simulink model "leftshift"  (R2024a)
settings: Solver=VariableStepAuto  StartTime=0.0  StopTime=10.0  RelTol=1e-3
libraries: simulink_extras x5
settings Model: Creator=prath  LastModifiedBy=prath

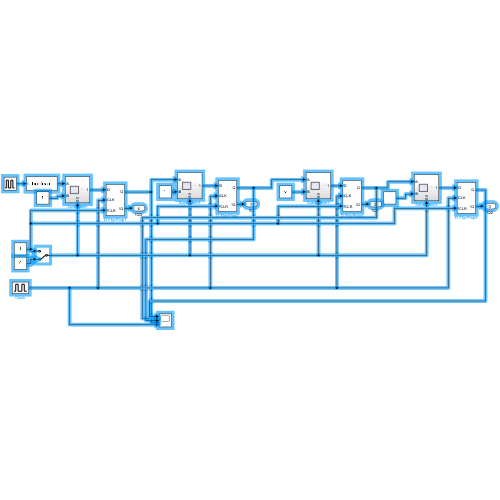
[thumbnail: Simulink's stored preview of the top-level diagram]
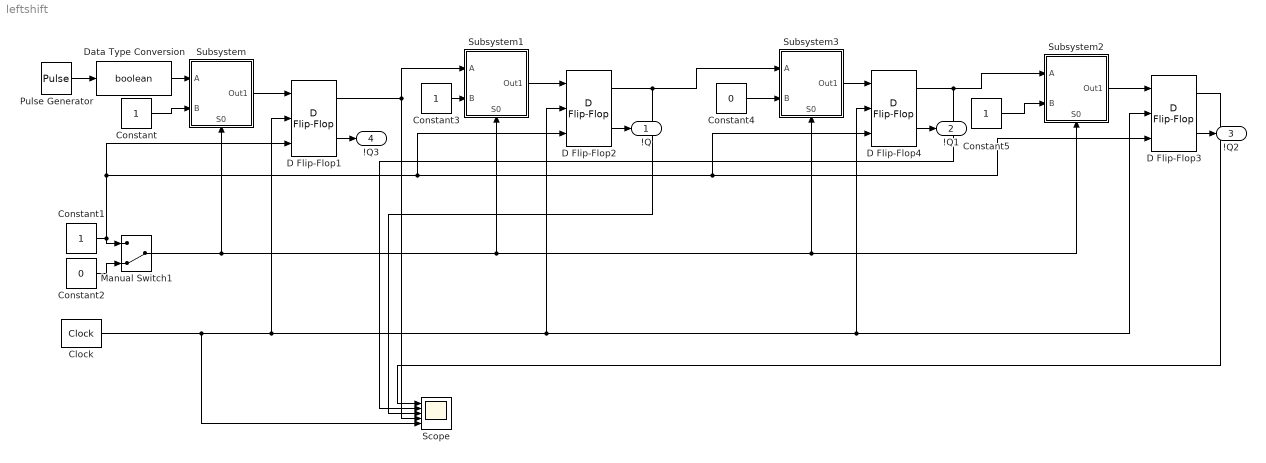
== system leftshift ==
  Clock : simulink_extras/Flip Flops/Clock  period=1
  Constant : Constant
  Constant1 : Constant  OutDataTypeStr=boolean
  Constant2 : Constant  Value=0  OutDataTypeStr=boolean
  Constant3 : Constant  OutDataTypeStr=boolean
  Constant4 : Constant  Value=0  OutDataTypeStr=boolean
  Constant5 : Constant  OutDataTypeStr=boolean
  D Flip-Flop{1..4} (4 alike) : simulink_extras/Flip Flops/D Flip-Flop
  Data Type Conversion : DataTypeConversion  OutDataTypeStr=boolean  SaturateOnIntegerOverflow=off  RndMeth=Floor
  Manual Switch1 : ManualSwitch  CurrentSetting=0
  Pulse Generator : DiscretePulseGenerator  PulseType=Time based  PulseWidth=50
  Scope : Scope  NumInputPorts=5
  Subsystem : Subsystem
      settings: PortSchema="{\"entries\":[{\"content\":{\"sides\":[{\"content\":{\"connectorIds\":[\"In1\",\"In2\"]},\"type\":\"ConnectorPlacement.EquallySpacedRectSide\",\"uuid\":\"2b5babe2-2f8b-4255-a93c-442313dac02f\"},{\"content\":{\"connectorIds\":[\"Out1\"],\"side\":\"RIGHT\"},\"type\":\"ConnectorPlacement.EquallySpacedRectSide\",\"uuid\":\"d00cf0b8-9821-435f-8e0a-21d3f86eeeec\"},{\"content\":{\"side\":\"TOP\"},\"type\":\"ConnectorPlacement.EquallySpacedRectSide\",\"uuid\":\"aded218e-ad72-4b70-8373-6f3260b36647\"},{\"content\":{\"connectorIds\":[\"In3\"],\"side\":\"BOTTOM\"},\"type\":\"ConnectorPlacement.EquallySpacedRectSide\",\"uuid\":\"ccb2f48e-c23e-4309-aab1-41b35e60905c\"}]},\"type\":\"ConnectorPlacement.EquallySpacedConnector\",\"uuid\":\"f3540823-2819-4903-8dd7-ac751c0ceac7\"}],\"packageUris\":[\"http://schema.mathworks.com/mf0/Connector/R2020b\"],\"version\":\"1.0\"}"
  Subsystem1 : Subsystem
      settings: PortSchema="{\"entries\":[{\"content\":{\"sides\":[{\"content\":{\"connectorIds\":[\"In1\",\"In2\"]},\"type\":\"ConnectorPlacement.EquallySpacedRectSide\",\"uuid\":\"2b5babe2-2f8b-4255-a93c-442313dac02f\"},{\"content\":{\"connectorIds\":[\"Out1\"],\"side\":\"RIGHT\"},\"type\":\"ConnectorPlacement.EquallySpacedRectSide\",\"uuid\":\"d00cf0b8-9821-435f-8e0a-21d3f86eeeec\"},{\"content\":{\"side\":\"TOP\"},\"type\":\"ConnectorPlacement.EquallySpacedRectSide\",\"uuid\":\"aded218e-ad72-4b70-8373-6f3260b36647\"},{\"content\":{\"connectorIds\":[\"In3\"],\"side\":\"BOTTOM\"},\"type\":\"ConnectorPlacement.EquallySpacedRectSide\",\"uuid\":\"ccb2f48e-c23e-4309-aab1-41b35e60905c\"}]},\"type\":\"ConnectorPlacement.EquallySpacedConnector\",\"uuid\":\"f3540823-2819-4903-8dd7-ac751c0ceac7\"}],\"packageUris\":[\"http://schema.mathworks.com/mf0/Connector/R2020b\"],\"version\":\"1.0\"}"
  Subsystem2 : Subsystem
      settings: PortSchema="{\"entries\":[{\"content\":{\"sides\":[{\"content\":{\"connectorIds\":[\"In1\",\"In2\"]},\"type\":\"ConnectorPlacement.EquallySpacedRectSide\",\"uuid\":\"2b5babe2-2f8b-4255-a93c-442313dac02f\"},{\"content\":{\"connectorIds\":[\"Out1\"],\"side\":\"RIGHT\"},\"type\":\"ConnectorPlacement.EquallySpacedRectSide\",\"uuid\":\"d00cf0b8-9821-435f-8e0a-21d3f86eeeec\"},{\"content\":{\"side\":\"TOP\"},\"type\":\"ConnectorPlacement.EquallySpacedRectSide\",\"uuid\":\"aded218e-ad72-4b70-8373-6f3260b36647\"},{\"content\":{\"connectorIds\":[\"In3\"],\"side\":\"BOTTOM\"},\"type\":\"ConnectorPlacement.EquallySpacedRectSide\",\"uuid\":\"ccb2f48e-c23e-4309-aab1-41b35e60905c\"}]},\"type\":\"ConnectorPlacement.EquallySpacedConnector\",\"uuid\":\"f3540823-2819-4903-8dd7-ac751c0ceac7\"}],\"packageUris\":[\"http://schema.mathworks.com/mf0/Connector/R2020b\"],\"version\":\"1.0\"}"
  Subsystem3 : Subsystem
      settings: PortSchema="{\"entries\":[{\"content\":{\"sides\":[{\"content\":{\"connectorIds\":[\"In1\",\"In2\"]},\"type\":\"ConnectorPlacement.EquallySpacedRectSide\",\"uuid\":\"2b5babe2-2f8b-4255-a93c-442313dac02f\"},{\"content\":{\"connectorIds\":[\"Out1\"],\"side\":\"RIGHT\"},\"type\":\"ConnectorPlacement.EquallySpacedRectSide\",\"uuid\":\"d00cf0b8-9821-435f-8e0a-21d3f86eeeec\"},{\"content\":{\"side\":\"TOP\"},\"type\":\"ConnectorPlacement.EquallySpacedRectSide\",\"uuid\":\"aded218e-ad72-4b70-8373-6f3260b36647\"},{\"content\":{\"connectorIds\":[\"In3\"],\"side\":\"BOTTOM\"},\"type\":\"ConnectorPlacement.EquallySpacedRectSide\",\"uuid\":\"ccb2f48e-c23e-4309-aab1-41b35e60905c\"}]},\"type\":\"ConnectorPlacement.EquallySpacedConnector\",\"uuid\":\"f3540823-2819-4903-8dd7-ac751c0ceac7\"}],\"packageUris\":[\"http://schema.mathworks.com/mf0/Connector/R2020b\"],\"version\":\"1.0\"}"
  !Q : Outport
  !Q1 : Outport  Port=2
  !Q2 : Outport  Port=3
  !Q3 : Outport  Port=4
  wires:
  D Flip-Flop1/2 -> !Q3/1
  D Flip-Flop3/2 -> !Q2/1
  D Flip-Flop4/1 -> Scope/2, Subsystem2/1(A)
  Constant4/1 -> Subsystem3/2(B)
  Clock/1 -> Scope/5, D Flip-Flop3/2, D Flip-Flop4/2, D Flip-Flop2/2, D Flip-Flop1/2
  D Flip-Flop4/2 -> !Q1/1
  Data Type Conversion/1 -> Subsystem/1(A)
  Subsystem1/1(Out1) -> D Flip-Flop2/1
  D Flip-Flop2/2 -> !Q/1
  D Flip-Flop1/1 -> Scope/4, Subsystem1/1(A)
  Subsystem2/1(Out1) -> D Flip-Flop3/1
  Constant3/1 -> Subsystem1/2(B)
  Subsystem3/1(Out1) -> D Flip-Flop4/1
  Pulse Generator/1 -> Data Type Conversion/1
  Constant/1 -> Subsystem/2(B)
  Manual Switch1/1 -> Subsystem2/3(S0), Subsystem3/3(S0), Subsystem1/3(S0), Subsystem/3(S0)
  Constant5/1 -> Subsystem2/2(B)
  D Flip-Flop2/1 -> Scope/3, Subsystem3/1(A)
  D Flip-Flop3/1 -> Scope/1
  Subsystem/1(Out1) -> D Flip-Flop1/1
  Constant1/1 -> D Flip-Flop3/3, D Flip-Flop4/3, D Flip-Flop2/3, D Flip-Flop1/3, Manual Switch1/1
  Constant2/1 -> Manual Switch1/2

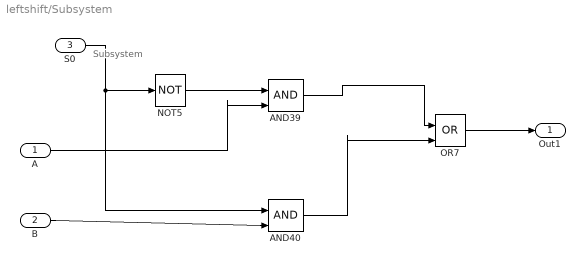
== system leftshift/Subsystem ==
  note: Subsystem
  A : Inport
  B : Inport  Port=2
  S0 : Inport  Port=3
  AND39 : Logic  IconShape=distinctive  AllPortsSameDT=off  OutDataTypeStr=boolean
  AND40 : Logic  IconShape=distinctive  AllPortsSameDT=off  OutDataTypeStr=boolean
  NOT5 : Logic  Operator=NOT  IconShape=distinctive  AllPortsSameDT=off  OutDataTypeStr=boolean
  OR7 : Logic  Operator=OR  IconShape=distinctive  AllPortsSameDT=off  OutDataTypeStr=boolean
  Out1 : Outport
  wires:
  A/1 -> AND39/2
  OR7/1 -> Out1/1
  S0/1 -> AND40/1, NOT5/1
  AND39/1 -> OR7/1
  NOT5/1 -> AND39/1
  B/1 -> AND40/2
  AND40/1 -> OR7/2

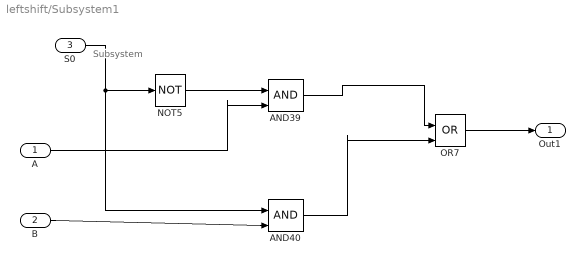
== system leftshift/Subsystem1 ==
  note: Subsystem
  A : Inport
  B : Inport  Port=2
  S0 : Inport  Port=3
  AND39 : Logic  IconShape=distinctive  AllPortsSameDT=off  OutDataTypeStr=boolean
  AND40 : Logic  IconShape=distinctive  AllPortsSameDT=off  OutDataTypeStr=boolean
  NOT5 : Logic  Operator=NOT  IconShape=distinctive  AllPortsSameDT=off  OutDataTypeStr=boolean
  OR7 : Logic  Operator=OR  IconShape=distinctive  AllPortsSameDT=off  OutDataTypeStr=boolean
  Out1 : Outport
  wires:
  A/1 -> AND39/2
  OR7/1 -> Out1/1
  S0/1 -> AND40/1, NOT5/1
  AND39/1 -> OR7/1
  NOT5/1 -> AND39/1
  B/1 -> AND40/2
  AND40/1 -> OR7/2

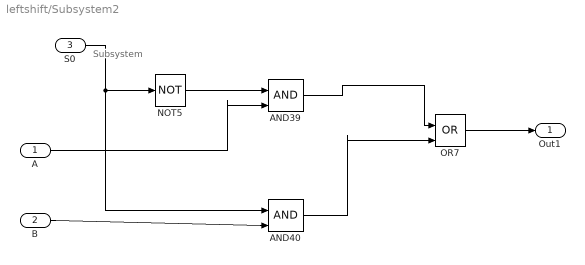
== system leftshift/Subsystem2 ==
  note: Subsystem
  A : Inport
  B : Inport  Port=2
  S0 : Inport  Port=3
  AND39 : Logic  IconShape=distinctive  AllPortsSameDT=off  OutDataTypeStr=boolean
  AND40 : Logic  IconShape=distinctive  AllPortsSameDT=off  OutDataTypeStr=boolean
  NOT5 : Logic  Operator=NOT  IconShape=distinctive  AllPortsSameDT=off  OutDataTypeStr=boolean
  OR7 : Logic  Operator=OR  IconShape=distinctive  AllPortsSameDT=off  OutDataTypeStr=boolean
  Out1 : Outport
  wires:
  A/1 -> AND39/2
  OR7/1 -> Out1/1
  S0/1 -> AND40/1, NOT5/1
  AND39/1 -> OR7/1
  NOT5/1 -> AND39/1
  B/1 -> AND40/2
  AND40/1 -> OR7/2

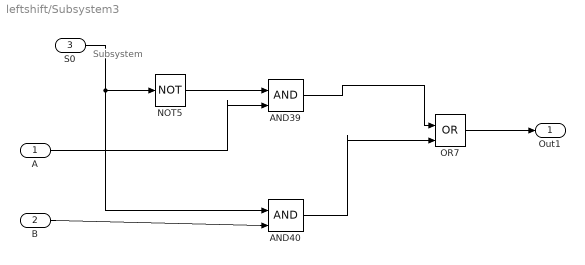
== system leftshift/Subsystem3 ==
  note: Subsystem
  A : Inport
  B : Inport  Port=2
  S0 : Inport  Port=3
  AND39 : Logic  IconShape=distinctive  AllPortsSameDT=off  OutDataTypeStr=boolean
  AND40 : Logic  IconShape=distinctive  AllPortsSameDT=off  OutDataTypeStr=boolean
  NOT5 : Logic  Operator=NOT  IconShape=distinctive  AllPortsSameDT=off  OutDataTypeStr=boolean
  OR7 : Logic  Operator=OR  IconShape=distinctive  AllPortsSameDT=off  OutDataTypeStr=boolean
  Out1 : Outport
  wires:
  AND40/1 -> OR7/2
  B/1 -> AND40/2
  NOT5/1 -> AND39/1
  AND39/1 -> OR7/1
  S0/1 -> NOT5/1, AND40/1
  OR7/1 -> Out1/1
  A/1 -> AND39/2
